simulink model "Quad_Controller"  (R2022b)
settings: Solver=ode4  StartTime=0.0  StopTime=20  FixedStep=0.01  RelTol=1e-3
InitFcn:
  | Initialize
StopFcn:
  | ending
values from neighbouring files (symbols this model uses):
  body =     [Initial_WorkSpace.mat]
  chi0 =     [Initial_WorkSpace.mat]
  g = 9.81    [Initial_WorkSpace.mat]    (also in Initialize.m)
  lambda0 =     [Initial_WorkSpace.mat]
  omega0 =     [Initial_WorkSpace.mat]
  s = tf('s')    [Initialize.m]
  v0 =     [Initial_WorkSpace.mat]
  wh = 250.367142553    [Initial_WorkSpace.mat]    (also in Initialize.m = sqrt(body.m*g/4/body.b))
undefined symbols (not defined in the file or in its folder): X, Y, Z
libraries: nesl_utility x22, sm_lib x17, simulink x5, sharedtransform x4, simulink_extras x3, matrix_library x2, uavutilslib x1
settings Model: Creator=Alire  LastModifiedBy=Alire

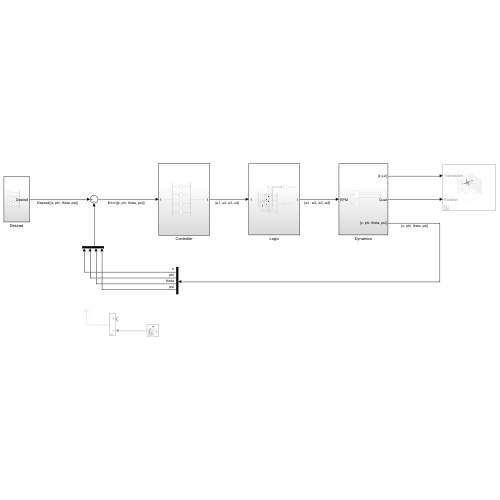
[thumbnail: Simulink's stored preview of the top-level diagram]
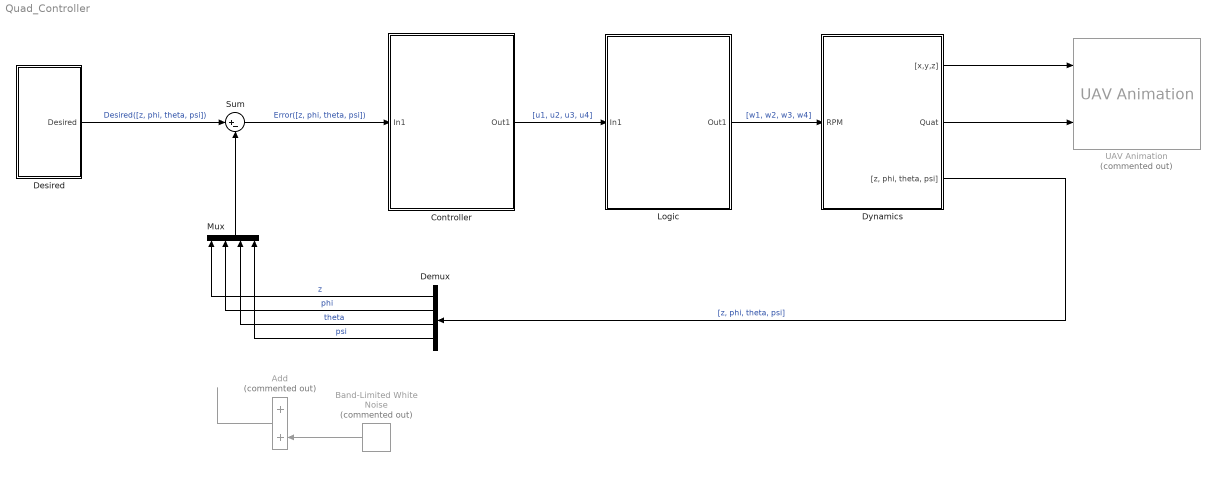
== system Quad_Controller ==
  Add : Sum  Commented=on
  Band-Limited White Noise : simulink/Sources/Band-Limited White Noise  Commented=on  Cov=[0.5*(pi/180)]  Ts=0.1  seed=[23341]
  Controller : Subsystem
  Demux : Demux
  Desired : Subsystem
  Dynamics : Subsystem
  Logic : Subsystem
  Mux : Mux
  Sum : Sum  Inputs=|+-
  UAV Animation : uavutilslib/UAV Animation  Commented=on  UAVType=Multirotor  UAVSize=10  InertialZDirection=Down  SampleTime=-1
  wires:
  Desired/1(Desired) -> Sum/1  "Desired([z, phi, theta, psi])"
  Sum/1 -> Controller/1(In1)  "Error([z, phi, theta, psi])"
  Controller/1(Out1) -> Logic/1(In1)  "[u1, u2, u3, u4]"
  Logic/1(Out1) -> Dynamics/1(RPM)  "[w1, w2, w3, w4]"
  Dynamics/3("[z, phi, theta, psi]") -> Demux/1  "[z, phi, theta, psi]"
  Dynamics/1("[x,y,z]") -> UAV Animation/1
  Dynamics/2(Quat) -> UAV Animation/2
  Mux/1 -> Sum/2
  Demux/1 -> Mux/1  "z"
  Demux/2 -> Mux/2  "phi"
  Demux/3 -> Mux/3  "theta"
  Demux/4 -> Mux/4  "psi"
  Band-Limited White Noise/1 -> Add/2
  Add/1 -> ?

== system Quad_Controller/Controller ==
  In1 : Inport
  Demux : Demux
  Gc_phi : Subsystem
  Gc_psi : Subsystem
  Gc_theta : Subsystem
  Gc_z : Subsystem
  Mux : Mux
  Out1 : Outport
  wires:
  In1/1 -> Demux/1
  Mux/1 -> Out1/1
  Demux/1 -> Gc_z/1(In1)
  Gc_z/1(u1) -> Mux/1
  Demux/2 -> Gc_phi/1(In1)
  Demux/3 -> Gc_theta/1(In1)
  Gc_theta/1(u3) -> Mux/3
  Gc_psi/1(u4) -> Mux/4
  Demux/4 -> Gc_psi/1(In1)
  Gc_phi/1(u2) -> Mux/2

== system Quad_Controller/Desired ==
  Degrees to Radians : simulink_extras/Transformations/Degrees to Radians
  Degrees to Radians1 : simulink_extras/Transformations/Degrees to Radians
  Degrees to Radians2 : simulink_extras/Transformations/Degrees to Radians
  Mux : Mux
  Z_desired : Constant  Value=-1
  phi_desired : Constant  Value=0
  psi_desired : Constant  Value=8
  theta_desired : Constant  Value=0
  Desired : Outport
  wires:
  Z_desired/1 -> Mux/1
  Mux/1 -> Desired/1
  theta_desired/1 -> Degrees to Radians1/1
  phi_desired/1 -> Degrees to Radians/1
  psi_desired/1 -> Degrees to Radians2/1
  Degrees to Radians/1 -> Mux/2
  Degrees to Radians1/1 -> Mux/3
  Degrees to Radians2/1 -> Mux/4

== system Quad_Controller/Dynamics ==
  RPM : Inport
  Phase1_Model : Subsystem
  Phase3_Model : Subsystem  Commented=on
  "[x,y,z]" : Outport
  Quat : Outport  Port=2
  "[z, phi, theta, psi]" : Outport  Port=3
  wires:
  RPM/1 -> Phase3_Model/1(rpm), Phase1_Model/1(RPM)
  Phase1_Model/1(x,y,z) -> "[x,y,z]"/1
  Phase1_Model/2(Quat) -> Quat/1
  Phase1_Model/3("[z, lambda]") -> "[z, phi, theta, psi]"/1

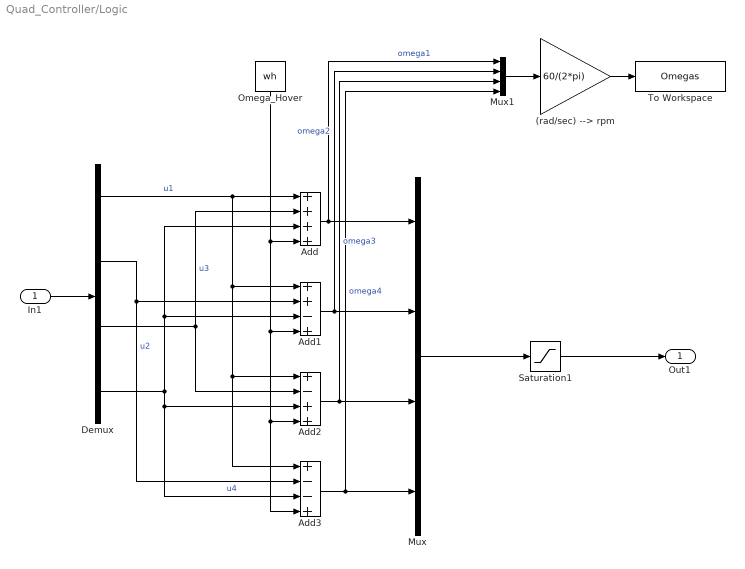
== system Quad_Controller/Logic ==
  In1 : Inport
  (rad/sec) --> rpm : Gain  Gain=60/(2*pi)
  Add : Sum  Inputs=++++
  Add1 : Sum  Inputs=++-+
  Add2 : Sum  Inputs=+-++
  Add3 : Sum  Inputs=+--+
  Demux : Demux
  Mux : Mux
  Mux1 : Mux
  Omega_Hover : Constant  Value=wh
  Saturation1 : Saturate  UpperLimit=350  LowerLimit=-200
  To Workspace : ToWorkspace  VariableName=Omegas  SampleTime=-1
  Out1 : Outport
  wires:
  In1/1 -> Demux/1
  Demux/1 -> Add/1, Add3/1, Add2/1, Add1/1  "u1"
  Demux/2 -> Add3/2, Add1/2  "u2"
  Demux/3 -> Add2/2, Add/2  "u3"
  Demux/4 -> Add2/3, Add3/3, Add1/3, Add/3  "u4"
  Add/1 -> Mux/1, Mux1/1  "omega1"
  Add1/1 -> Mux/2, Mux1/2  "omega2"
  Add2/1 -> Mux/3, Mux1/3  "omega3"
  Add3/1 -> Mux/4, Mux1/4  "omega4"
  Mux/1 -> Saturation1/1
  Omega_Hover/1 -> Add/4, Add3/4, Add2/4, Add1/4
  Mux1/1 -> (rad/sec) --> rpm/1
  (rad/sec) --> rpm/1 -> To Workspace/1
  Saturation1/1 -> Out1/1

== system Quad_Controller/Controller/Gc_phi ==
  In1 : Inport
  Add : Sum
  Derivative : Derivative
  Gain : Gain  Gain=8.7e3
  Gain1 : Gain  Gain=450
  u2 : Outport
  wires:
  Gain1/1 -> Derivative/1
  Gain/1 -> Add/1
  Add/1 -> u2/1  "u2"
  Derivative/1 -> Add/2
  In1/1 -> Gain/1, Gain1/1

== system Quad_Controller/Controller/Gc_psi ==
  In1 : Inport
  Add : Sum
  Derivative : Derivative
  Gain : Gain  Gain=12.5e3
  Gain1 : Gain  Gain=650
  u4 : Outport
  wires:
  Gain1/1 -> Derivative/1
  Gain/1 -> Add/1
  Add/1 -> u4/1  "u4"
  Derivative/1 -> Add/2
  In1/1 -> Gain1/1, Gain/1

== system Quad_Controller/Controller/Gc_theta ==
  In1 : Inport
  Add : Sum
  Derivative : Derivative
  Gain : Gain  Gain=8.6e3
  Gain1 : Gain  Gain=445
  u3 : Outport
  wires:
  In1/1 -> Gain1/1, Gain/1
  Derivative/1 -> Add/2
  Add/1 -> u3/1  "u3"
  Gain/1 -> Add/1
  Gain1/1 -> Derivative/1

== system Quad_Controller/Controller/Gc_z ==
  In1 : Inport
  Add : Sum
  Derivative : Derivative
  Gain : Gain  Gain=-38e3
  Gain1 : Gain  Gain=-20e3
  u1 : Outport
  wires:
  In1/1 -> Gain1/1, Gain/1
  Derivative/1 -> Add/2
  Add/1 -> u1/1  "u1"
  Gain/1 -> Add/1
  Gain1/1 -> Derivative/1

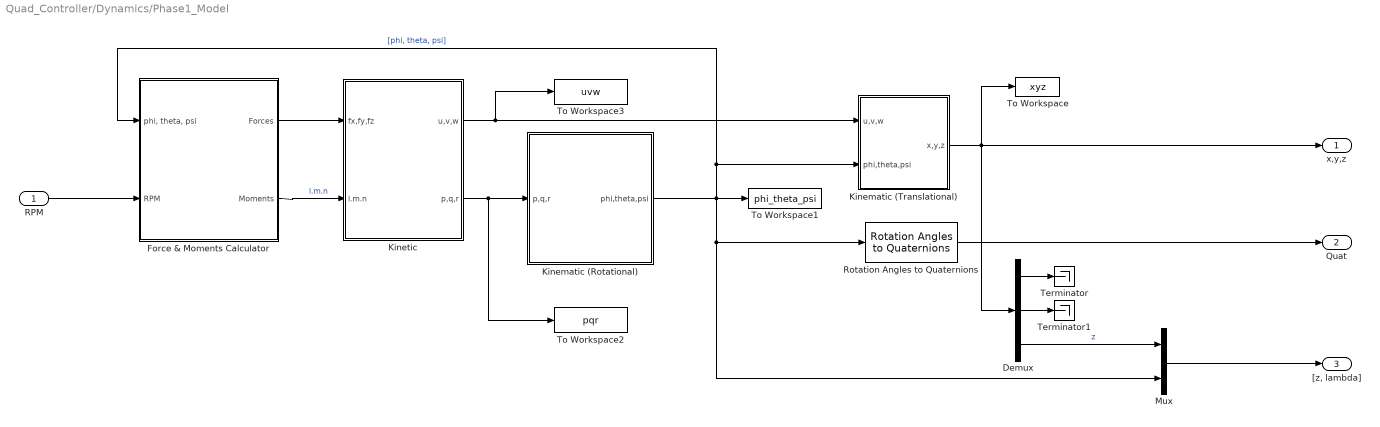
== system Quad_Controller/Dynamics/Phase1_Model ==
  RPM : Inport
  Demux : Demux  Outputs=3
  Force & Moments Calculator : Subsystem
  Kinematic (Rotational) : Subsystem
  Kinematic (Translational) : Subsystem
  Kinetic : Subsystem
  Mux : Mux  Inputs=2
  Rotation Angles to Quaternions : sharedtransform/Rotation Angles to Quaternions  rotationOrder=ZYX  aMode=aMode
  Terminator : Terminator
  Terminator1 : Terminator
  To Workspace : ToWorkspace  VariableName=xyz  SampleTime=-1
  To Workspace1 : ToWorkspace  VariableName=phi_theta_psi  SampleTime=-1
  To Workspace2 : ToWorkspace  VariableName=pqr  SampleTime=-1
  To Workspace3 : ToWorkspace  VariableName=uvw  SampleTime=-1
  x,y,z : Outport
  Quat : Outport  Port=2
  "[z, lambda]" : Outport  Port=3
  wires:
  Kinetic/1(u,v,w) -> Kinematic (Translational)/1(u,v,w), To Workspace3/1
  Kinetic/2(p,q,r) -> To Workspace2/1, Kinematic (Rotational)/1(p,q,r)
  Demux/3 -> Mux/1  "z"
  Force & Moments Calculator/1(Forces) -> Kinetic/1(fx,fy,fz)
  RPM/1 -> Force & Moments Calculator/2(RPM)
  Kinematic (Translational)/1(x,y,z) -> x,y,z/1, Demux/1, To Workspace/1
  Force & Moments Calculator/2(Moments) -> Kinetic/2(l.m.n)  "l.m.n"
  Demux/2 -> Terminator1/1
  Demux/1 -> Terminator/1
  Rotation Angles to Quaternions/1 -> Quat/1
  Kinematic (Rotational)/1(phi,theta,psi) -> Force & Moments Calculator/1("phi, theta, psi"), Kinematic (Translational)/2(phi,theta,psi), Mux/2, Rotation Angles to Quaternions/1, To Workspace1/1  "[phi, theta, psi]"
  Mux/1 -> "[z, lambda]"/1

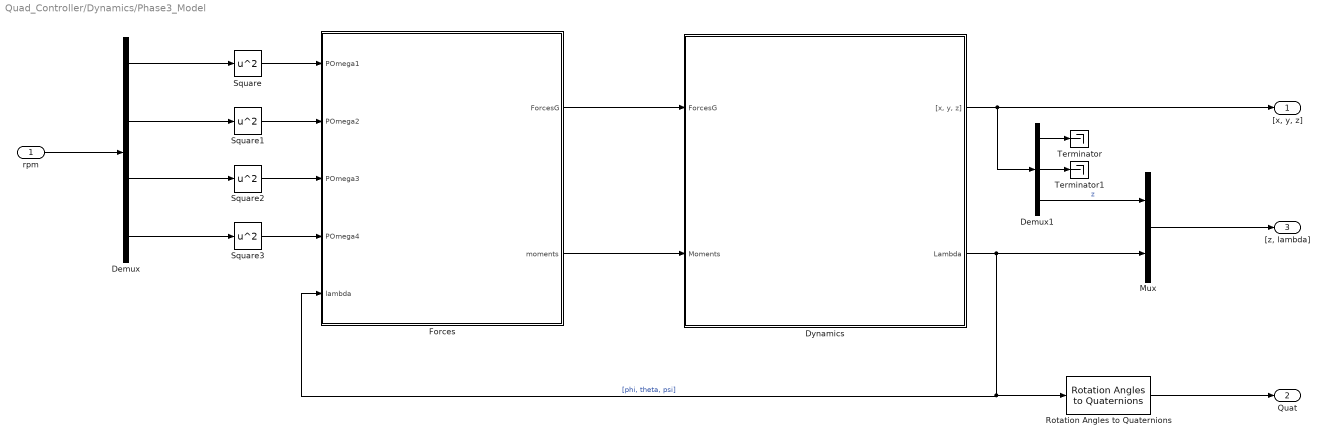
== system Quad_Controller/Dynamics/Phase3_Model ==
  rpm : Inport
  Demux : Demux
  Demux1 : Demux  Outputs=3
  Dynamics : Subsystem
  Forces : Subsystem
  Mux : Mux  Inputs=2
  Rotation Angles to Quaternions : sharedtransform/Rotation Angles to Quaternions  rotationOrder=ZYX  aMode=aMode
  Square{,1..3} (4 alike) : Math  Operator=square
  Terminator : Terminator
  Terminator1 : Terminator
  "[x, y, z]" : Outport
  Quat : Outport  Port=2
  "[z, lambda]" : Outport  Port=3
  wires:
  Demux/1 -> Square/1
  Dynamics/2(Lambda) -> Forces/5(lambda), Rotation Angles to Quaternions/1, Mux/2  "[phi, theta, psi]"
  Square2/1 -> Forces/3(POmega3)
  Square/1 -> Forces/1(POmega1)
  Demux/3 -> Square2/1
  Square1/1 -> Forces/2(POmega2)
  Square3/1 -> Forces/4(POmega4)
  Demux/4 -> Square3/1
  Demux/2 -> Square1/1
  Forces/1(ForcesG) -> Dynamics/1(ForcesG)
  Forces/2(moments) -> Dynamics/2(Moments)
  rpm/1 -> Demux/1
  Mux/1 -> "[z, lambda]"/1
  Demux1/2 -> Terminator1/1
  Demux1/3 -> Mux/1  "z"
  Demux1/1 -> Terminator/1
  Dynamics/1("[x, y, z]") -> "[x, y, z]"/1, Demux1/1
  Rotation Angles to Quaternions/1 -> Quat/1

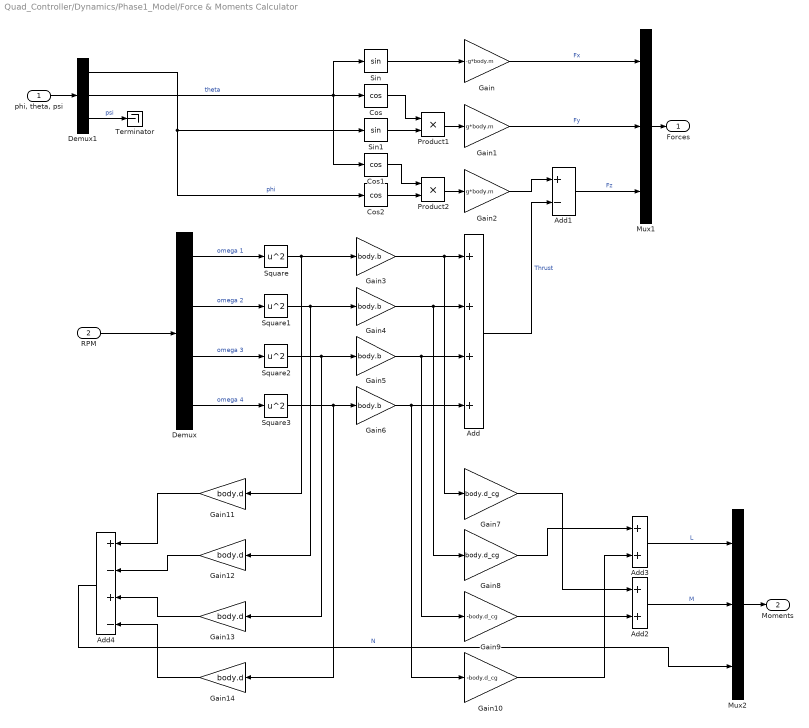
== system Quad_Controller/Dynamics/Phase1_Model/Force & Moments Calculator ==
  "phi, theta, psi" : Inport
  RPM : Inport  Port=2
  Add : Sum  Inputs=++++
  Add1 : Sum  Inputs=+-
  Add2 : Sum
  Add3 : Sum
  Add4 : Sum  Inputs=+-+-
  Cos : Trigonometry  Operator=cos
  Cos1 : Trigonometry  Operator=cos
  Cos2 : Trigonometry  Operator=cos
  Demux : Demux
  Demux1 : Demux  Outputs=3
  Gain : Gain  Gain=-g*body.m
  Gain1 : Gain  Gain=g*body.m
  Gain10 : Gain  Gain=-body.d_cg
  Gain{11..14} (4 alike) : Gain  Gain=body.d
  Gain2 : Gain  Gain=g*body.m
  Gain{3..6} (4 alike) : Gain  Gain=body.b
  Gain7 : Gain  Gain=body.d_cg
  Gain8 : Gain  Gain=body.d_cg
  Gain9 : Gain  Gain=-body.d_cg
  Mux1 : Mux  Inputs=3
  Mux2 : Mux  Inputs=3
  Product1 : Product
  Product2 : Product
  Sin : Trigonometry
  Sin1 : Trigonometry
  Square{,1..3} (4 alike) : Math  Operator=square
  Terminator : Terminator
  Forces : Outport
  Moments : Outport  Port=2
  wires:
  Cos2/1 -> Product2/2
  Cos1/1 -> Product2/1
  Gain1/1 -> Mux1/2  "Fy"
  Demux/3 -> Square2/1  "omega 3"
  Gain5/1 -> Gain9/1, Add/3
  Gain2/1 -> Add1/1
  Demux1/1 -> Sin1/1, Cos2/1  "phi"
  Add3/1 -> Mux2/1  "L"
  Gain4/1 -> Gain8/1, Add/2
  Gain6/1 -> Gain10/1, Add/4
  Gain3/1 -> Gain7/1, Add/1
  Demux/2 -> Square1/1  "omega 2"
  Gain9/1 -> Add2/2
  Sin1/1 -> Product1/2
  Gain/1 -> Mux1/1  "Fx"
  Add2/1 -> Mux2/2  "M"
  Gain13/1 -> Add4/3
  Demux/1 -> Square/1  "omega 1"
  Square2/1 -> Gain13/1, Gain5/1
  Demux1/2 -> Sin/1, Cos1/1, Cos/1  "theta"
  Gain7/1 -> Add2/1
  Gain14/1 -> Add4/4
  Demux/4 -> Square3/1  "omega 4"
  Cos/1 -> Product1/1
  Gain12/1 -> Add4/2
  Square3/1 -> Gain14/1, Gain6/1
  Add/1 -> Add1/2  "Thrust"
  Add4/1 -> Mux2/3  "N"
  Mux2/1 -> Moments/1
  Gain11/1 -> Add4/1
  Sin/1 -> Gain/1
  Product1/1 -> Gain1/1
  Add1/1 -> Mux1/3  "Fz"
  Gain8/1 -> Add3/1
  RPM/1 -> Demux/1
  Square1/1 -> Gain12/1, Gain4/1
  Square/1 -> Gain11/1, Gain3/1
  Gain10/1 -> Add3/2
  Product2/1 -> Gain2/1
  Mux1/1 -> Forces/1
  "phi, theta, psi"/1 -> Demux1/1
  Demux1/3 -> Terminator/1  "psi"

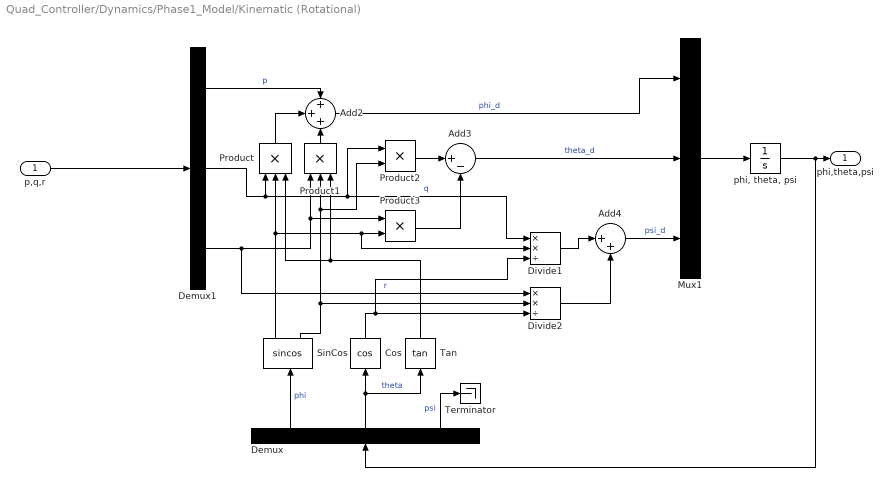
== system Quad_Controller/Dynamics/Phase1_Model/Kinematic (Rotational) ==
  p,q,r : Inport
  Add2 : Sum  Inputs=+++
  Add3 : Sum  Inputs=|+-
  Add4 : Sum  Inputs=|++
  Cos : Trigonometry  Operator=cos
  Demux : Demux  Outputs=3
  Demux1 : Demux  Outputs=3
  Divide1 : Product  Inputs=**/
  Divide2 : Product  Inputs=**/
  Mux1 : Mux  Inputs=3
  Product : Product  Inputs=3
  Product1 : Product  Inputs=3
  Product2 : Product
  Product3 : Product
  SinCos : Trigonometry  Operator=sincos
  Tan : Trigonometry  Operator=tan
  Terminator : Terminator
  "phi, theta, psi" : Integrator  InitialCondition=[lambda0.phi, lambda0.theta, lambda0.psi]
  phi,theta,psi : Outport
  wires:
  SinCos/2 -> Divide2/2, Product2/2, Product1/2
  Divide1/1 -> Add4/1
  Product1/1 -> Add2/3
  Demux1/2 -> Product/1, Divide1/1, Product2/1  "q"
  Demux1/3 -> Divide2/1, Product3/1, Product1/1  "r"
  Product2/1 -> Add3/1
  Tan/1 -> Product1/3, Product/3
  Demux/3 -> Terminator/1  "psi"
  Mux1/1 -> "phi, theta, psi"/1
  Cos/1 -> Divide2/3, Divide1/3
  Demux/1 -> SinCos/1  "phi"
  SinCos/1 -> Divide1/2, Product3/2, Product/2
  Add2/1 -> Mux1/1  "phi_d"
  Demux1/1 -> Add2/1  "p"
  Product/1 -> Add2/2
  Demux/2 -> Cos/1, Tan/1  "theta"
  Product3/1 -> Add3/2
  Add3/1 -> Mux1/2  "theta_d"
  Add4/1 -> Mux1/3  "psi_d"
  Divide2/1 -> Add4/2
  "phi, theta, psi"/1 -> Demux/1, phi,theta,psi/1
  p,q,r/1 -> Demux1/1

== system Quad_Controller/Dynamics/Phase1_Model/Kinematic (Translational) ==
  u,v,w : Inport
  phi,theta,psi : Inport  Port=2
  MatrixMultiply2 : Product  Multiplication=Matrix(*)
  Rotation Angles to Direction Cosine Matrix : sharedtransform/Rotation Angles to Direction Cosine Matrix  rotationOrder=ZYX  aMode=aMode
  Selector9 : Selector  InputPortWidth=3  IndexOptions=Index vector (dialog)  Indices=[3 2 1]  OutputSizes=1
  Transpose : Math  Operator=transpose
  "x, y, z" : Integrator  InitialCondition=[chi0.x, chi0.y, chi0.z]
  x,y,z : Outport
  wires:
  Transpose/1 -> MatrixMultiply2/1
  Selector9/1 -> Rotation Angles to Direction Cosine Matrix/1
  MatrixMultiply2/1 -> "x, y, z"/1
  u,v,w/1 -> MatrixMultiply2/2
  Rotation Angles to Direction Cosine Matrix/1 -> Transpose/1
  "x, y, z"/1 -> x,y,z/1
  phi,theta,psi/1 -> Selector9/1

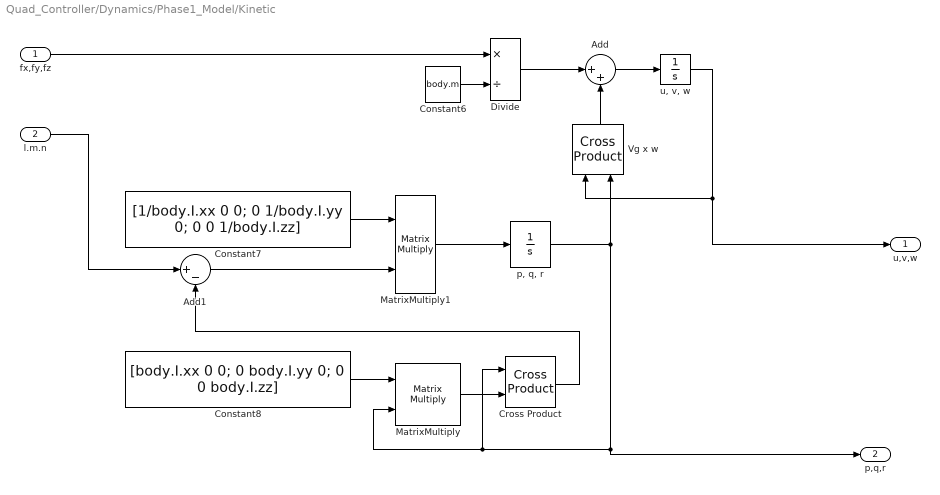
== system Quad_Controller/Dynamics/Phase1_Model/Kinetic ==
  fx,fy,fz : Inport
  l.m.n : Inport  Port=2
  Add : Sum  Inputs=|++
  Add1 : Sum  Inputs=|+-
  Constant6 : Constant  Value=body.m
  Constant7 : Constant  Value="[1/body.I.xx 0 0; 0 1/body.I.yy 0; 0 0  1/body.I.zz]"
  Constant8 : Constant  Value="[body.I.xx 0 0; 0 body.I.yy 0; 0 0  body.I.zz]"
  Cross Product : matrix_library/Cross Product
  Divide : Product  Inputs=*/
  MatrixMultiply : Product  Multiplication=Matrix(*)
  MatrixMultiply1 : Product  Multiplication=Matrix(*)
  Vg x w : matrix_library/Cross Product
  "p, q, r" : Integrator  InitialCondition=[omega0.p, omega0.q, omega0.r]
  "u, v, w" : Integrator  InitialCondition=[v0.x, v0.y, v0.z]
  u,v,w : Outport
  p,q,r : Outport  Port=2
  wires:
  "u, v, w"/1 -> u,v,w/1, Vg x w/1
  Vg x w/1 -> Add/2
  Constant6/1 -> Divide/2
  Add1/1 -> MatrixMultiply1/2
  "p, q, r"/1 -> p,q,r/1, Cross Product/1, MatrixMultiply/2, Vg x w/2
  Divide/1 -> Add/1
  Constant8/1 -> MatrixMultiply/1
  Add/1 -> "u, v, w"/1
  Cross Product/1 -> Add1/2
  MatrixMultiply/1 -> Cross Product/2
  Constant7/1 -> MatrixMultiply1/1
  fx,fy,fz/1 -> Divide/1
  MatrixMultiply1/1 -> "p, q, r"/1
  l.m.n/1 -> Add1/1

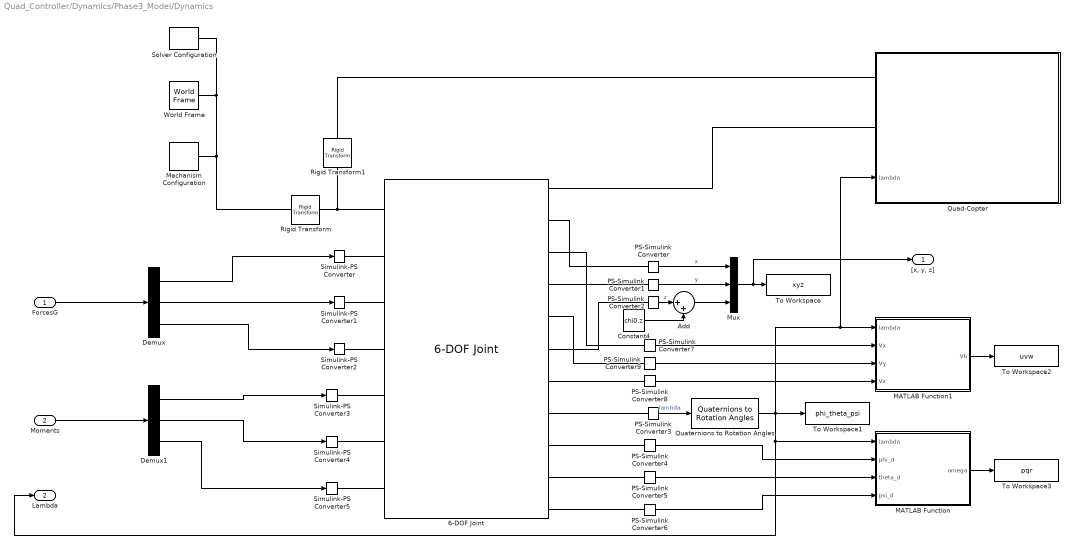
== system Quad_Controller/Dynamics/Phase3_Model/Dynamics ==
  ForcesG : Inport
  Moments : Inport  Port=2
  6-DOF Joint : sm_lib/Joints/6-DOF Joint  JointMode=Normal  SenseConstraintForce=off  SenseConstraintForceX=off  SenseConstraintForceY=off  SenseConstraintForceZ=off  SenseConstraintTorque=off  SenseConstraintTorqueX=off  SenseConstraintTorqueY=off  SenseConstraintTorqueZ=off  SenseTotalForce=off  SenseTotalForceX=off  SenseTotalForceY=off  SenseTotalForceZ=off  SenseTotalTorque=off  SenseTotalTorqueX=off  SenseTotalTorqueY=off  SenseTotalTorqueZ=off  CompositeWrenchDir=FollowerOnBase  CompositeWrenchFrame=BaseFrame  PxEquilibriumPosition=0  PxEquilibriumPositionUnits=m  PxSpringStiffness=0  PxSpringStiffnessUnits=N/m  PxDampingCoefficient=0  PxDampingCoefficientUnits=N/(m/s)  PxTorqueActuationMode=InputTorque  PxMotionActuationMode=ComputedMotion  PxSensePosition=on  PxSenseVelocity=on  PxSenseAcceleration=off  PxSenseTorqueForce=off  PxSenseLowerLimitTorqueForce=off  PxSenseUpperLimitTorqueForce=off  PxLowerLimitSpecify=off  PxLowerLimitBound=-1  PxLowerLimitBoundUnits=m  PxLowerLimitStiffness=1e6  PxLowerLimitStiffnessUnits=N/m  PxLowerLimitDamping=1e3  PxLowerLimitDampingUnits=N/(m/s)  PxLowerLimitTransitionRegionWidth=1e-4  PxLowerLimitTransitionRegionWidthUnits=m  PxUpperLimitSpecify=off  PxUpperLimitBound=1  PxUpperLimitBoundUnits=m  PxUpperLimitStiffness=1e6  PxUpperLimitStiffnessUnits=N/m  PxUpperLimitDamping=1e3  PxUpperLimitDampingUnits=N/(m/s)  PxUpperLimitTransitionRegionWidth=1e-4  PxUpperLimitTransitionRegionWidthUnits=m  PxPositionTargetSpecify=off  PxPositionTargetPriority=High  PxPositionTargetValue=0  PxPositionTargetValueUnits=m  PxVelocityTargetSpecify=off  PxVelocityTargetPriority=High  PxVelocityTargetValue=0  PxVelocityTargetValueUnits=m/s  PyEquilibriumPosition=0  PyEquilibriumPositionUnits=m  PySpringStiffness=0  PySpringStiffnessUnits=N/m  PyDampingCoefficient=0  PyDampingCoefficientUnits=N/(m/s)  PyTorqueActuationMode=InputTorque  PyMotionActuationMode=ComputedMotion  PySensePosition=on  PySenseVelocity=on  PySenseAcceleration=off  PySenseTorqueForce=off  PySenseLowerLimitTorqueForce=off  PySenseUpperLimitTorqueForce=off  PyLowerLimitSpecify=off  PyLowerLimitBound=-1  PyLowerLimitBoundUnits=m  PyLowerLimitStiffness=1e6  PyLowerLimitStiffnessUnits=N/m  PyLowerLimitDamping=1e3  PyLowerLimitDampingUnits=N/(m/s)  PyLowerLimitTransitionRegionWidth=1e-4  PyLowerLimitTransitionRegionWidthUnits=m  PyUpperLimitSpecify=off  PyUpperLimitBound=1  PyUpperLimitBoundUnits=m  PyUpperLimitStiffness=1e6  PyUpperLimitStiffnessUnits=N/m  PyUpperLimitDamping=1e3  PyUpperLimitDampingUnits=N/(m/s)  PyUpperLimitTransitionRegionWidth=1e-4  PyUpperLimitTransitionRegionWidthUnits=m  PyPositionTargetSpecify=off  PyPositionTargetPriority=High  PyPositionTargetValue=0  PyPositionTargetValueUnits=m  PyVelocityTargetSpecify=off  PyVelocityTargetPriority=High  PyVelocityTargetValue=0  PyVelocityTargetValueUnits=m/s  PzEquilibriumPosition=0  PzEquilibriumPositionUnits=m  PzSpringStiffness=0  PzSpringStiffnessUnits=N/m  PzDampingCoefficient=0  PzDampingCoefficientUnits=N/(m/s)  PzTorqueActuationMode=InputTorque  PzMotionActuationMode=ComputedMotion  PzSensePosition=on  PzSenseVelocity=on  PzSenseAcceleration=off  PzSenseTorqueForce=off  PzSenseLowerLimitTorqueForce=off  PzSenseUpperLimitTorqueForce=off  PzLowerLimitSpecify=off  PzLowerLimitBound=-1  PzLowerLimitBoundUnits=m  PzLowerLimitStiffness=1e6  PzLowerLimitStiffnessUnits=N/m  PzLowerLimitDamping=1e3  PzLowerLimitDampingUnits=N/(m/s)  PzLowerLimitTransitionRegionWidth=1e-4  PzLowerLimitTransitionRegionWidthUnits=m  PzUpperLimitSpecify=off  PzUpperLimitBound=1  PzUpperLimitBoundUnits=m  PzUpperLimitStiffness=1e6  PzUpperLimitStiffnessUnits=N/m  PzUpperLimitDamping=1e3  PzUpperLimitDampingUnits=N/(m/s)  PzUpperLimitTransitionRegionWidth=1e-4  PzUpperLimitTransitionRegionWidthUnits=m  PzPositionTargetSpecify=off  PzPositionTargetPriority=High  PzPositionTargetValue=0  PzPositionTargetValueUnits=m  PzVelocityTargetSpecify=off  PzVelocityTargetPriority=High  PzVelocityTargetValue=0  PzVelocityTargetValueUnits=m/s  SphEqPosRotationMethod=None  SphEqPosRotationAngleUnits=deg  SphEqPosRotationStandardAxis=+Z  SphEqPosRotationAngle=0.0  SphEqPosRotationArbitraryAxis=[0 0 1]  SphEqPosFollAlignAxisA=+X  SphEqPosBaseAlignAxisA=+Y  SphEqPosFollAlignAxisB=+Y  SphEqPosBaseAlignAxisB=+Z  SphEqPosRotationSequenceAxes=FollowerAxes  SphEqPosRotationSequence=XYX  SphEqPosRotationSequenceAngles=[0 0 0]  SphEqPosRotationSequenceAnglesUnits=deg  SphEqPosRotationMatrix=[1 0 0; 0 1 0; 0 0 1]  SphEqPosQuaternion=[1 0 0 0]  SphSpringStiffness=0  SphSpringStiffnessUnits=N*m/deg  SphDampingCoefficient=0  SphDampingCoefficientUnits=N*m/(deg/s)  SphActuateTorqueX=on  SphActuateTorqueY=on  SphActuateTorqueZ=on  SphActuateTorque=off  SphTorqueActuationMode=InputTorque  SphMotionActuationMode=ComputedMotion  SphActuationFrame=BaseFrame  SphSensePosition=on  SphSenseVelocityX=on  SphSenseVelocityY=on  SphSenseVelocityZ=on  SphSenseVelocity=off  SphSenseAccelerationX=off  SphSenseAccelerationY=off  SphSenseAccelerationZ=off  SphSenseAcceleration=off  SphSenseTorqueX=off  SphSenseTorqueY=off  SphSenseTorqueZ=off  SphSenseTorqueForce=off  SphSenseLowerLimitTorqueMag=off  SphSenseUpperLimitTorqueMag=off  SphSensingFrame=BaseFrame  SphLowerLimitSpecify=off  SphLowerLimitBound=15  SphLowerLimitBoundUnits=deg  SphLowerLimitStiffness=1e4  SphLowerLimitStiffnessUnits=N*m/deg  SphLowerLimitDamping=10  SphLowerLimitDampingUnits=N*m/(deg/s)  SphLowerLimitTransitionRegionWidth=0.1  SphLowerLimitTransitionRegionWidthUnits=deg  SphUpperLimitSpecify=off  SphUpperLimitBound=45  SphUpperLimitBoundUnits=deg  SphUpperLimitStiffness=1e4  SphUpperLimitStiffnessUnits=N*m/deg  SphUpperLimitDamping=10  SphUpperLimitDampingUnits=N*m/(deg/s)  SphUpperLimitTransitionRegionWidth=0.1  SphUpperLimitTransitionRegionWidthUnits=deg  SphPositionTargetRotationMethod=None  SphPositionTargetRotationAngleUnits=deg  SphPositionTargetRotationStandardAxis=+Z  SphPositionTargetRotationAngle=0.0  SphPositionTargetRotationArbitraryAxis=[0 0 1]  SphPositionTargetFollAlignAxisA=+X  SphPositionTargetBaseAlignAxisA=+Y  SphPositionTargetFollAlignAxisB=+Y  SphPositionTargetBaseAlignAxisB=+Z  SphPositionTargetRotationSequenceAxes=FollowerAxes  SphPositionTargetRotationSequence=XYX  SphPositionTargetRotationSequenceAngles=[0 0 0]  SphPositionTargetRotationSequenceAnglesUnits=deg  SphPositionTargetRotationMatrix=[1 0 0; 0 1 0; 0 0 1]  SphPositionTargetQuaternion=[1 0 0 0]  SphPositionTargetSpecify=off  SphPositionTargetPriority=High  SphVelocityTargetValue=[0 0 0]  SphVelocityTargetValueUnits=deg/s  SphVelocityTargetSpecify=off  SphVelocityTargetPriority=High  SphVelocityTargetInFollowerFrame=on
  Add : Sum  Inputs=|++
  Constant4 : Constant  Value=chi0.z
  Demux : Demux  Outputs=3
  Demux1 : Demux  Outputs=3
  MATLAB Function : MATLAB Function  TreatAsAtomicUnit=on
  MATLAB Function1 : MATLAB Function  TreatAsAtomicUnit=on
  Mechanism Configuration : sm_lib/Utilities/Mechanism Configuration  UniformGravity=Constant  GravityVector=[0 0 -9.81]  GravityUnits=m/s^2  LinearizationDelta=0.001  JointModeTransitionNonlinearIterations=2
  Mux : Mux  Inputs=3
  PS-Simulink Converter{,1..9} (10 alike) : nesl_utility/PS-Simulink Converter  PhysicalDomain=network_engine_domain  SubClassName=ps_output  LeftPortType=input  RightPortType=output  PseudoPeriodic=off  Frequencies=[]  VectorFormat=inherit  Unit=inherit  AffineConversion=off
  Quad-Copter : Subsystem
      settings: PortSchema="{\"entries\":[{\"content\":{\"sides\":[{\"content\":{\"connectorIds\":[\"LConn1\",\"LConn2\",\"In1\"]},\"type\":\"ConnectorPlacement.EquallySpacedRectSide\",\"uuid\":\"04743956-a569-41a7-b22c-bd483dcea0b7\"},{\"content\":{\"connectorIds\":[],\"side\":\"RIGHT\"},\"type\":\"ConnectorPlacement.EquallySpacedRectSide\",\"uuid\":\"9bc8017a-87dc-4fac-922f-a31a079728db\"},{\"content\":{\"connectorIds\":[],\"side\":\"TOP\"},\"type\":\"ConnectorPlacement.EquallySpacedRectSide\",\"uuid\":\"e9bdb144-97c5-4666-a0dc-c713dd3d3caa\"}]},\"type\":\"ConnectorPlacement.EquallySpacedConnector\",\"uuid\":\"315c4317-d40d-4cb5-b79a-0df11d629229\"}],\"packageUris\":[\"http://schema.mathworks.com/mf0/Connector/R2020b\"],\"version\":\"1.0\"}"
  Quaternions to Rotation Angles : sharedtransform/Quaternions to Rotation Angles  rotationOrder=XYZ  aMode=aMode
  Rigid Transform : sm_lib/Frames and Transforms/Rigid Transform  TranslationMethod=None  TranslationStandardOffset=0  TranslationLengthUnit=m  TranslationStandardAxis=+Z  TranslationCartesianOffset=[0 0 0]  TranslationROffset=0  TranslationROffsetUnits=m  TranslationZOffset=0  TranslationZOffsetUnits=m  TranslationThetaOffset=0  TranslationThetaOffsetUnits=deg  RotationMethod=StandardAxis  RotationAngleUnits=deg  RotationStandardAxis=+X  RotationAngle=180  RotationArbitraryAxis=[0 0 1]  FollAlignAxisA=+X  BaseAlignAxisA=+Y  FollAlignAxisB=+Y  BaseAlignAxisB=+Z  RotationSequenceAxes=FollowerAxes  RotationSequence=XYX  RotationSequenceAngles=[0 0 0]  RotationSequenceAnglesUnits=deg  RotationMatrix=[1 0 0; 0 1 0; 0 0 1]  Quaternion=[1 0 0 0]
  Rigid Transform1 : sm_lib/Frames and Transforms/Rigid Transform  TranslationMethod=StandardAxis  TranslationStandardOffset=1  TranslationLengthUnit=m  TranslationStandardAxis=+Z  TranslationCartesianOffset=[0 0 0]  TranslationROffset=0  TranslationROffsetUnits=m  TranslationZOffset=0  TranslationZOffsetUnits=m  TranslationThetaOffset=0  TranslationThetaOffsetUnits=deg  RotationMethod=None  RotationAngleUnits=deg  RotationStandardAxis=+X  RotationAngle=180  RotationArbitraryAxis=[0 0 1]  FollAlignAxisA=+X  BaseAlignAxisA=+Y  FollAlignAxisB=+Y  BaseAlignAxisB=+Z  RotationSequenceAxes=FollowerAxes  RotationSequence=XYX  RotationSequenceAngles=[0 0 0]  RotationSequenceAnglesUnits=deg  RotationMatrix=[1 0 0; 0 1 0; 0 0 1]  Quaternion=[1 0 0 0]
  Simulink-PS Converter{,1..5} (6 alike) : nesl_utility/Simulink-PS Converter  PhysicalDomain=network_engine_domain  SubClassName=ps_input  LeftPortType=input  RightPortType=output  PseudoPeriodic=off  Frequencies=[]  NoiseDistribution=none  NoiseParameters=[]  Unit=1  AffineConversion=off  FilteringAndDerivatives=provide  SimscapeFilterOrder=1  InputFilterTimeConstant=0.001  UdotUserProvided=0
  Solver Configuration : nesl_utility/Solver Configuration  PhysicalDomain=network_engine_domain  SubClassName=solver  LeftPortType=input  RightPortType=generic  Tones=[]  Harmonics=[]  SimulateNoise=off  Profile=off  UseLocalSampling=off  EnableSwitchedLinearOptims=on  FrequencyDomain=off  UseCCode=off  RelTol=0.001  AbsTol=1e-06  MinStep=1e-09  ToWorkspace=off  RevertToSquareIcSolve=off  NumHomotopyIterations=100  PhasorMode=off  PhasorModeNumHarmonics=1  ConsistencySolver=NEWTON_XTOL_AFTER_FTOL  IndexReductionMethod=DerivativeReplacement  DoDC=off  ResidualTolerance=1e-09  ConsistencyTolSource=GLOBAL  ConsistencyAbsTol=0.001  ConsistencyRelTol=0.001  ConsistencyTolFactor=0.001  UseLocalSolver=off  LocalSolverChoice=NE_BACKWARD_EULER_ADVANCER  ResolveIndetEquations=on  FunctionEvalNumThread=1  LocalSolverSampleTime=0.001  DoFixedCost=off  MaxNonlinIter=3  MaxModeIter=2  ComputeImpulses=off  ImpulseIterations=2  LinearAlgebra=Sparse  LinearAlgebraNumThread=0  EquationFormulation=NE_TIME_EF  DelaysMemoryBudget=1024  AutomaticFiltering=on  FilteringTimeConstant=0.001  PartitionStorageMethod=AS_NEEDED  PartitionMemoryBudget=1024  PartitionMethod=FAST
  To Workspace : ToWorkspace  VariableName=xyz  SampleTime=-1
      settings: Save2DSignal=2-D array (concatenate along first dimension)
  To Workspace1 : ToWorkspace  VariableName=phi_theta_psi  SampleTime=-1
      settings: Save2DSignal=2-D array (concatenate along first dimension)
  To Workspace2 : ToWorkspace  VariableName=uvw  SampleTime=-1
      settings: Save2DSignal=2-D array (concatenate along first dimension)
  To Workspace3 : ToWorkspace  VariableName=pqr  SampleTime=-1
      settings: Save2DSignal=2-D array (concatenate along first dimension)
  World Frame : sm_lib/Frames and Transforms/World Frame
  "[x, y, z]" : Outport
  Lambda : Outport  Port=2
  wires:
  PS-Simulink Converter/1 -> Mux/1  "x"
  PS-Simulink Converter9/1 -> MATLAB Function1/3(Vy)
  Add/1 -> Mux/3
  Demux/2 -> Simulink-PS Converter1/1
  PS-Simulink Converter2/1 -> Add/1  "z"
  Quaternions to Rotation Angles/1 -> Quad-Copter/1(lambda), MATLAB Function1/1(lambda), Lambda/1, MATLAB Function/1(lambda), To Workspace1/1
  Demux1/1 -> Simulink-PS Converter3/1
  Demux/3 -> Simulink-PS Converter2/1
  ForcesG/1 -> Demux/1
  PS-Simulink Converter1/1 -> Mux/2  "y"
  PS-Simulink Converter8/1 -> MATLAB Function1/4(Vz)
  Demux1/3 -> Simulink-PS Converter5/1
  PS-Simulink Converter5/1 -> MATLAB Function/3(theta_d)
  Demux1/2 -> Simulink-PS Converter4/1
  Constant4/1 -> Add/2
  Demux/1 -> Simulink-PS Converter/1
  Mux/1 -> "[x, y, z]"/1, To Workspace/1
  MATLAB Function/1(omega) -> To Workspace3/1
  PS-Simulink Converter4/1 -> MATLAB Function/2(phi_d)
  PS-Simulink Converter3/1 -> Quaternions to Rotation Angles/1  "lambda"
  MATLAB Function1/1(Vb) -> To Workspace2/1
  PS-Simulink Converter7/1 -> MATLAB Function1/2(Vx)
  PS-Simulink Converter6/1 -> MATLAB Function/4(psi_d)
  Moments/1 -> Demux1/1
  connections:
  Rigid Transform/RConn1 -- 6-DOF Joint/LConn1 -- Rigid Transform1/LConn1
  Simulink-PS Converter1/RConn1 -- 6-DOF Joint/LConn3
  6-DOF Joint/RConn2 -- PS-Simulink Converter/LConn1
  Simulink-PS Converter2/RConn1 -- 6-DOF Joint/LConn4
  PS-Simulink Converter1/LConn1 -- 6-DOF Joint/RConn4
  6-DOF Joint/RConn11 -- PS-Simulink Converter6/LConn1
  6-DOF Joint/RConn8 -- PS-Simulink Converter3/LConn1
  6-DOF Joint/RConn6 -- PS-Simulink Converter2/LConn1
  6-DOF Joint/RConn10 -- PS-Simulink Converter5/LConn1
  6-DOF Joint/RConn5 -- PS-Simulink Converter9/LConn1
  Mechanism Configuration/RConn1 -- Rigid Transform/LConn1 -- World Frame/RConn1 -- Solver Configuration/RConn1
  Simulink-PS Converter5/RConn1 -- 6-DOF Joint/LConn7
  Simulink-PS Converter/RConn1 -- 6-DOF Joint/LConn2
  Simulink-PS Converter4/RConn1 -- 6-DOF Joint/LConn6
  6-DOF Joint/RConn7 -- PS-Simulink Converter8/LConn1
  Simulink-PS Converter3/RConn1 -- 6-DOF Joint/LConn5
  6-DOF Joint/RConn9 -- PS-Simulink Converter4/LConn1
  6-DOF Joint/RConn3 -- PS-Simulink Converter7/LConn1
  Quad-Copter/LConn2 -- 6-DOF Joint/RConn1
  Rigid Transform1/RConn1 -- Quad-Copter/LConn1

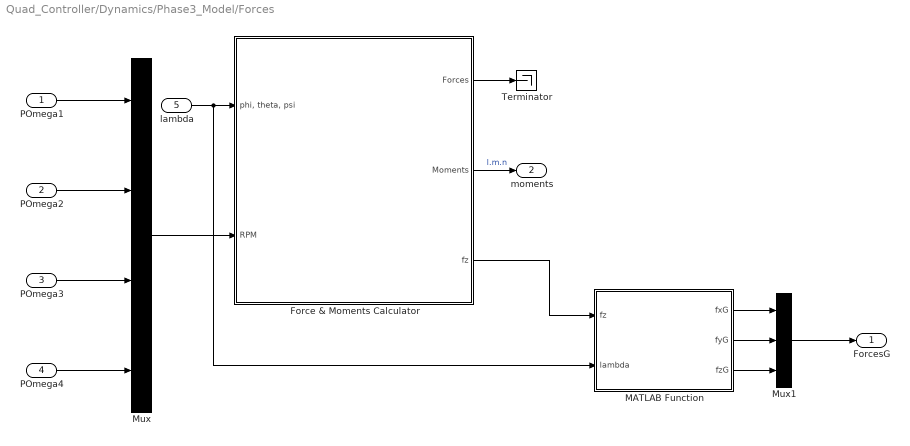
== system Quad_Controller/Dynamics/Phase3_Model/Forces ==
  POmega1 : Inport
  POmega2 : Inport  Port=2
  POmega3 : Inport  Port=3
  POmega4 : Inport  Port=4
  lambda : Inport  Port=5
  Force & Moments Calculator : Subsystem
  MATLAB Function : MATLAB Function  TreatAsAtomicUnit=on
  Mux : Mux
  Mux1 : Mux  Inputs=3
  Terminator : Terminator
  ForcesG : Outport
  moments : Outport  Port=2
  wires:
  Force & Moments Calculator/2(Moments) -> moments/1  "l.m.n"
  POmega3/1 -> Mux/3
  POmega1/1 -> Mux/1
  Mux/1 -> Force & Moments Calculator/2(RPM)
  POmega4/1 -> Mux/4
  POmega2/1 -> Mux/2
  lambda/1 -> MATLAB Function/2(lambda), Force & Moments Calculator/1("phi, theta, psi")
  Force & Moments Calculator/3(fz) -> MATLAB Function/1(fz)
  MATLAB Function/1(fxG) -> Mux1/1
  MATLAB Function/2(fyG) -> Mux1/2
  MATLAB Function/3(fzG) -> Mux1/3
  Mux1/1 -> ForcesG/1
  Force & Moments Calculator/1(Forces) -> Terminator/1

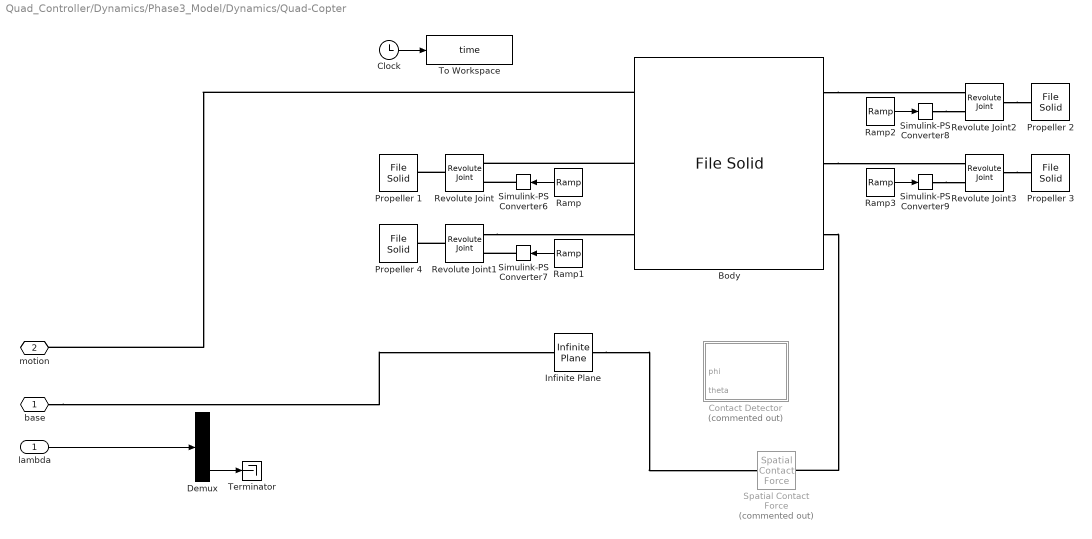
== system Quad_Controller/Dynamics/Phase3_Model/Dynamics/Quad-Copter ==
  lambda : Inport
  Body : sm_lib/Body Elements/File Solid  ExtGeomFileName=SolidFiles\body.STEP  UnitType=FromFile  ExtGeomFileUnits=m  StepReaderType=HEX  ExportConvexHullGeometry=on  InertiaType=Custom  Mass=0.8  MassUnits=kg  CenterOfMass=[-333.85 324.3 -438.13]  CenterOfMassUnits=mm  MomentsOfInertia=[0.02839 0.03066 0.04390]  MomentsOfInertiaUnits=kg*m^2  ProductsOfInertia=[0 0 0]  ProductsOfInertiaUnits=kg*m^2  BasedOnType=DensityFromFile  Density=1000  DensityUnits=kg/m^3  DoExposeReferenceFrame=off  SerializedFrames=<Frames><Frame><Id>Frame1</Id><Value><Name>CG</Name><Origin><Source>CenterOfMassFrame</Source><FeatureName></FeatureName></Origin><PrimaryAxis><DefinedDirection>+Z</DefinedDirection><Source>ReferenceFrame</Source><SourceDirection>+Z</SourceDirection><FeatureName></FeatureName></PrimaryAxis><SecondaryAxis><DefinedDirection>+X</DefinedDirection><Source>ReferenceFrame</Source><SourceDirection>+X</SourceDirection><FeatureName></FeatureName></SecondaryAxis></Value></Frame><Frame><Id>Frame2</Id><Value><Name>M2</Name><Origin><Source>GeometricFeature</Source><FeatureName>circular curve 838</FeatureName></Origin><PrimaryAxis><DefinedDirection>+Z</DefinedDirection><Source>ReferenceFrame</Source><SourceDirection>+Z</SourceDirection><FeatureName></FeatureName></PrimaryAxis><SecondaryAxis><DefinedDirection>+X</DefinedDirection><Source>ReferenceFrame</Source><SourceDirection>+X</SourceDirection><FeatureName></FeatureName></SecondaryAxis></Value></Frame><Frame><Id>Frame3</Id><Value><Name>M1</Name><Origin><Source>GeometricFeature</Source><FeatureName>circular curve 1634</FeatureName></Origin><PrimaryAxis><DefinedDirection>+Z</DefinedDirection><Source>ReferenceFrame</Source><SourceDirection>+Z</SourceDirection><FeatureName></FeatureName></PrimaryAxis><SecondaryAxis><DefinedDirection>+Y</DefinedDirection><Source>ReferenceFrame</Source><SourceDirection>+X</SourceDirection><FeatureName></FeatureName></SecondaryAxis></Value></Frame><Frame><Id>Frame4</Id><Value><Name>M3</Name><Origin><Source>GeometricFeature</Source><FeatureName>circular curve 1236</FeatureName></Origin><PrimaryAxis><DefinedDirection>+Z</DefinedDirection><Source>ReferenceFrame</Source><SourceDirection>+Z</SourceDirection><FeatureName></FeatureName></PrimaryAxis><SecondaryAxis><DefinedDirection>+X</DefinedDirection><Source>ReferenceFrame</Source><SourceDirection>+X</SourceDirection><FeatureName></FeatureName></SecondaryAxis></Value></Frame><Frame><Id>Frame5</Id><Value><Name>M4</Name><Origin><Source>GeometricFeature</Source><FeatureName>circular curve 2038</FeatureName></Origin><PrimaryAxis><DefinedDirection>+Z</DefinedDirection><Source>ReferenceFrame</Source><SourceDirection>+Z</SourceDirection><FeatureName></FeatureName></PrimaryAxis><SecondaryAxis><DefinedDirection>+X</DefinedDirection><Source>ReferenceFrame</Source><SourceDirection>+X</SourceDirection><FeatureName></FeatureName></SecondaryAxis></Value></Frame></Frames>  GraphicType=FromGeometry  MarkerShape=Sphere  MarkerSize=10  GraphicVisPropType=SimpleVisualProperties  GraphicDiffuseColor=[0.5 0.5 0.5]  GraphicSpecularColor=[0.5 0.5 0.5 1.0]  GraphicAmbientColor=[0.15 0.15 0.15 1.0]  GraphicEmissiveColor=[0.0 0.0 0.0 1.0]  GraphicShininess=75  GraphicOpacity=1.0
  Clock : Clock
  Contact Detector : Subsystem  Commented=on
      settings: PortSchema="{\"entries\":[{\"content\":{\"sides\":[{\"content\":{\"connectorIds\":[\"LConn1\",\"In1\",\"In2\"]},\"type\":\"ConnectorPlacement.EquallySpacedRectSide\",\"uuid\":\"73a6758d-74b0-4dfa-ae59-8f1544b47e52\"},{\"content\":{\"connectorIds\":[\"RConn1\"],\"side\":\"RIGHT\"},\"type\":\"ConnectorPlacement.EquallySpacedRectSide\",\"uuid\":\"cda79cee-8790-4a48-af2a-c8e672ccd871\"},{\"content\":{\"connectorIds\":[],\"side\":\"TOP\"},\"type\":\"ConnectorPlacement.EquallySpacedRectSide\",\"uuid\":\"3568e893-e479-4ecf-b205-b5b750c24788\"}]},\"type\":\"ConnectorPlacement.EquallySpacedConnector\",\"uuid\":\"7addec4e-c0c3-4372-b547-1236ed1106f4\"}],\"packageUris\":[\"http://schema.mathworks.com/mf0/Connector/R2020b\"],\"version\":\"1.0\"}"
  Demux : Demux  Outputs=3
  Infinite Plane : sm_lib/Curves and Surfaces/Infinite Plane  GraphicType=Rectangle  GraphicPlaneWidth=10  GraphicPlaneWidthUnits=m  GraphicPlaneHeight=10  GraphicPlaneHeightUnits=m  GraphicVisPropType=SimpleVisualProperties  GraphicDiffuseColor=[1 0.07451 0.651]  GraphicOpacity=0.25  GraphicSpecularColor=[0.5 0.5 0.5 1.0]  GraphicAmbientColor=[0.15 0.15 0.15 1.0]  GraphicEmissiveColor=[0.0 0.0 0.0 1.0]  GraphicShininess=75
  "Propeller 1 " : sm_lib/Body Elements/File Solid  ExtGeomFileName=SolidFiles\propeller_blade_black.STEP  UnitType=FromFile  ExtGeomFileUnits=m  StepReaderType=HEX  ExportConvexHullGeometry=off  InertiaType=Custom  Mass=0.00001  MassUnits=kg  CenterOfMass=[0 0 0]  CenterOfMassUnits=m  MomentsOfInertia=[1e-12 1e-12 1e-12]  MomentsOfInertiaUnits=kg*m^2  ProductsOfInertia=[0 0 0]  ProductsOfInertiaUnits=kg*m^2  BasedOnType=Mass  Density=1000  DensityUnits=kg/m^3  DoExposeReferenceFrame=off  SerializedFrames=<Frames><Frame><Id>Frame1</Id><Value><Name>F1</Name><Origin><Source>CenterOfMassFrame</Source><FeatureName></FeatureName></Origin><PrimaryAxis><DefinedDirection>-X</DefinedDirection><Source>ReferenceFrame</Source><SourceDirection>+Z</SourceDirection><FeatureName></FeatureName></PrimaryAxis><SecondaryAxis><DefinedDirection>+Y</DefinedDirection><Source>ReferenceFrame</Source><SourceDirection>+X</SourceDirection><FeatureName></FeatureName></SecondaryAxis></Value></Frame></Frames>  GraphicType=FromGeometry  MarkerShape=Sphere  MarkerSize=10  GraphicVisPropType=SimpleVisualProperties  GraphicDiffuseColor=[1.0 0.2 0.2]  GraphicSpecularColor=[0.5 0.5 0.5 1.0]  GraphicAmbientColor=[0.15 0.15 0.15 1.0]  GraphicEmissiveColor=[0.0 0.0 0.0 1.0]  GraphicShininess=75  GraphicOpacity=1.0
  Propeller 2 : sm_lib/Body Elements/File Solid  ExtGeomFileName=SolidFiles\propeller_blade_black.STEP  UnitType=FromFile  ExtGeomFileUnits=m  StepReaderType=HEX  ExportConvexHullGeometry=off  InertiaType=Custom  Mass=0.00001  MassUnits=kg  CenterOfMass=[0 0 0]  CenterOfMassUnits=m  MomentsOfInertia=[1e-12 1e-12 1e-12]  MomentsOfInertiaUnits=kg*m^2  ProductsOfInertia=[0 0 0]  ProductsOfInertiaUnits=kg*m^2  BasedOnType=Mass  Density=1000  DensityUnits=kg/m^3  DoExposeReferenceFrame=off  SerializedFrames=<Frames><Frame><Id>Frame1</Id><Value><Name>F1</Name><Origin><Source>CenterOfMassFrame</Source><FeatureName></FeatureName></Origin><PrimaryAxis><DefinedDirection>-X</DefinedDirection><Source>ReferenceFrame</Source><SourceDirection>+Z</SourceDirection><FeatureName></FeatureName></PrimaryAxis><SecondaryAxis><DefinedDirection>+Y</DefinedDirection><Source>ReferenceFrame</Source><SourceDirection>+X</SourceDirection><FeatureName></FeatureName></SecondaryAxis></Value></Frame></Frames>  GraphicType=FromGeometry  MarkerShape=Sphere  MarkerSize=10  GraphicVisPropType=SimpleVisualProperties  GraphicDiffuseColor=[1.0 0.2 0.2]  GraphicSpecularColor=[0.5 0.5 0.5 1.0]  GraphicAmbientColor=[0.15 0.15 0.15 1.0]  GraphicEmissiveColor=[0.0 0.0 0.0 1.0]  GraphicShininess=75  GraphicOpacity=1.0
  Propeller 3 : sm_lib/Body Elements/File Solid  ExtGeomFileName=SolidFiles\propeller_blade_black.STEP  UnitType=FromFile  ExtGeomFileUnits=m  StepReaderType=HEX  ExportConvexHullGeometry=off  InertiaType=Custom  Mass=0.00001  MassUnits=kg  CenterOfMass=[0 0 0]  CenterOfMassUnits=m  MomentsOfInertia=[1e-12 1e-12 1e-12]  MomentsOfInertiaUnits=kg*m^2  ProductsOfInertia=[0 0 0]  ProductsOfInertiaUnits=kg*m^2  BasedOnType=Mass  Density=1000  DensityUnits=kg/m^3  DoExposeReferenceFrame=off  SerializedFrames=<Frames><Frame><Id>Frame1</Id><Value><Name>F1</Name><Origin><Source>CenterOfMassFrame</Source><FeatureName></FeatureName></Origin><PrimaryAxis><DefinedDirection>-X</DefinedDirection><Source>ReferenceFrame</Source><SourceDirection>+Z</SourceDirection><FeatureName></FeatureName></PrimaryAxis><SecondaryAxis><DefinedDirection>+Y</DefinedDirection><Source>ReferenceFrame</Source><SourceDirection>+X</SourceDirection><FeatureName></FeatureName></SecondaryAxis></Value></Frame></Frames>  GraphicType=FromGeometry  MarkerShape=Sphere  MarkerSize=10  GraphicVisPropType=SimpleVisualProperties  GraphicDiffuseColor=[1.0 0.2 0.2]  GraphicSpecularColor=[0.5 0.5 0.5 1.0]  GraphicAmbientColor=[0.15 0.15 0.15 1.0]  GraphicEmissiveColor=[0.0 0.0 0.0 1.0]  GraphicShininess=75  GraphicOpacity=1.0
  Propeller 4 : sm_lib/Body Elements/File Solid  ExtGeomFileName=SolidFiles\propeller_blade_black.STEP  UnitType=FromFile  ExtGeomFileUnits=m  StepReaderType=HEX  ExportConvexHullGeometry=off  InertiaType=Custom  Mass=0.00001  MassUnits=kg  CenterOfMass=[0 0 0]  CenterOfMassUnits=m  MomentsOfInertia=[1e-12 1e-12 1e-12]  MomentsOfInertiaUnits=kg*m^2  ProductsOfInertia=[0 0 0]  ProductsOfInertiaUnits=kg*m^2  BasedOnType=Mass  Density=1000  DensityUnits=kg/m^3  DoExposeReferenceFrame=off  SerializedFrames=<Frames><Frame><Id>Frame1</Id><Value><Name>F1</Name><Origin><Source>CenterOfMassFrame</Source><FeatureName></FeatureName></Origin><PrimaryAxis><DefinedDirection>-X</DefinedDirection><Source>ReferenceFrame</Source><SourceDirection>+Z</SourceDirection><FeatureName></FeatureName></PrimaryAxis><SecondaryAxis><DefinedDirection>+Y</DefinedDirection><Source>ReferenceFrame</Source><SourceDirection>+X</SourceDirection><FeatureName></FeatureName></SecondaryAxis></Value></Frame></Frames>  GraphicType=FromGeometry  MarkerShape=Sphere  MarkerSize=10  GraphicVisPropType=SimpleVisualProperties  GraphicDiffuseColor=[1.0 0.2 0.2]  GraphicSpecularColor=[0.5 0.5 0.5 1.0]  GraphicAmbientColor=[0.15 0.15 0.15 1.0]  GraphicEmissiveColor=[0.0 0.0 0.0 1.0]  GraphicShininess=75  GraphicOpacity=1.0
  Ramp : simulink/Sources/Ramp  slope=-8  start=0  InitialOutput=0
  Ramp1 : simulink/Sources/Ramp  slope=8  start=0  InitialOutput=0
  Ramp2 : simulink/Sources/Ramp  slope=8  start=0  InitialOutput=0
  Ramp3 : simulink/Sources/Ramp  slope=-8  start=0  InitialOutput=0
  Revolute Joint{,1..3} (4 alike) : sm_lib/Joints/Revolute Joint  JointMode=Normal  SenseConstraintForce=off  SenseConstraintForceX=off  SenseConstraintForceY=off  SenseConstraintForceZ=off  SenseConstraintTorque=off  SenseConstraintTorqueX=off  SenseConstraintTorqueY=off  SenseConstraintTorqueZ=off  SenseTotalForce=off  SenseTotalForceX=off  SenseTotalForceY=off  SenseTotalForceZ=off  SenseTotalTorque=off  SenseTotalTorqueX=off  SenseTotalTorqueY=off  SenseTotalTorqueZ=off  CompositeWrenchDir=FollowerOnBase  CompositeWrenchFrame=BaseFrame  EquilibriumPosition=0  EquilibriumPositionUnits=deg  SpringStiffness=0  SpringStiffnessUnits=N*m/deg  DampingCoefficient=0  DampingCoefficientUnits=N*m/(deg/s)  TorqueActuationMode=ComputedTorque  MotionActuationMode=InputMotion  SensePosition=off  SenseVelocity=off  SenseAcceleration=off  SenseTorqueForce=off  SenseLowerLimitTorqueForce=off  SenseUpperLimitTorqueForce=off  LowerLimitSpecify=off  LowerLimitBound=-90  LowerLimitBoundUnits=deg  LowerLimitStiffness=1e4  LowerLimitStiffnessUnits=N*m/deg  LowerLimitDamping=10  LowerLimitDampingUnits=N*m/(deg/s)  LowerLimitTransitionRegionWidth=0.1  LowerLimitTransitionRegionWidthUnits=deg  UpperLimitSpecify=off  UpperLimitBound=90  UpperLimitBoundUnits=deg  UpperLimitStiffness=1e4  UpperLimitStiffnessUnits=N*m/deg  UpperLimitDamping=10  UpperLimitDampingUnits=N*m/(deg/s)  UpperLimitTransitionRegionWidth=0.1  UpperLimitTransitionRegionWidthUnits=deg  PositionTargetSpecify=off  PositionTargetPriority=High  PositionTargetValue=0  PositionTargetValueUnits=deg  VelocityTargetSpecify=off  VelocityTargetPriority=High  VelocityTargetValue=0  VelocityTargetValueUnits=deg/s
  Simulink-PS Converter{6..9} (4 alike) : nesl_utility/Simulink-PS Converter  PhysicalDomain=network_engine_domain  SubClassName=ps_input  LeftPortType=input  RightPortType=output  PseudoPeriodic=off  Frequencies=[]  NoiseDistribution=none  NoiseParameters=[]  Unit=1  AffineConversion=off  FilteringAndDerivatives=filter  SimscapeFilterOrder=2  InputFilterTimeConstant=0.1  UdotUserProvided=0
  Spatial Contact Force : sm_lib/Forces and Torques/Spatial Contact Force  Commented=on  SenseContactBaseRotation=off  SenseContactBaseTranslation=off  CoefficientOfDynamicFriction=0.3  CoefficientOfStaticFriction=0.5  NormalDamping=1e3  NormalDampingUnits=N/(m/s)  SenseContactSignal=off  NormalStiffness=1e6  NormalStiffnessUnits=N/m  FrictionalCriticalVelocity=1e-3  FrictionalCriticalVelocityUnits=m/s  ZeroCrossDetectContactStartAndEnd=off  SenseContactFollowerRotation=off  SenseContactFollowerTranslation=off  FrictionType=SmoothStickSlip  SenseFrictionalForceMagnitude=off  SenseNormalForceMagnitude=off  NormalForceType=SmoothSpringDamper  SenseNormalVelocity=off  SenseSeparationDistance=off  SenseTangentialVelocity=off  NormalTransitionRegionWidth=1e-4  NormalTransitionRegionWidthUnits=m
  Terminator : Terminator
  To Workspace : ToWorkspace  VariableName=time  SampleTime=-1
      settings: Save2DSignal=2-D array (concatenate along first dimension)
  base : PMIOPort  Side=Left
  motion : PMIOPort  Port=2  Side=Left
  wires:
  Ramp1/1 -> Simulink-PS Converter7/1
  Ramp3/1 -> Simulink-PS Converter9/1
  Ramp2/1 -> Simulink-PS Converter8/1
  Ramp/1 -> Simulink-PS Converter6/1
  Demux/3 -> Terminator/1
  lambda/1 -> Demux/1
  Clock/1 -> To Workspace/1
  connections:
  Simulink-PS Converter9/RConn1 -- Revolute Joint3/LConn2
  Simulink-PS Converter6/RConn1 -- Revolute Joint/LConn2
  Revolute Joint1/RConn1 -- Propeller 4/LConn1
  Simulink-PS Converter7/RConn1 -- Revolute Joint1/LConn2
  Revolute Joint1/LConn1 -- Body/LConn3
  Simulink-PS Converter8/RConn1 -- Revolute Joint2/LConn2
  Revolute Joint2/RConn1 -- Propeller 2/LConn1
  Body/LConn1 -- motion/RConn1
  Body/RConn2 -- Revolute Joint3/LConn1
  Body/LConn2 -- Revolute Joint/LConn1
  Body/RConn1 -- Revolute Joint2/LConn1
  Revolute Joint3/RConn1 -- Propeller 3/LConn1
  Revolute Joint/RConn1 -- "Propeller 1 "/LConn1
  base/RConn1 -- Infinite Plane/LConn1
  Body/RConn3 -- Spatial Contact Force/RConn1
  Infinite Plane/RConn1 -- Spatial Contact Force/LConn1

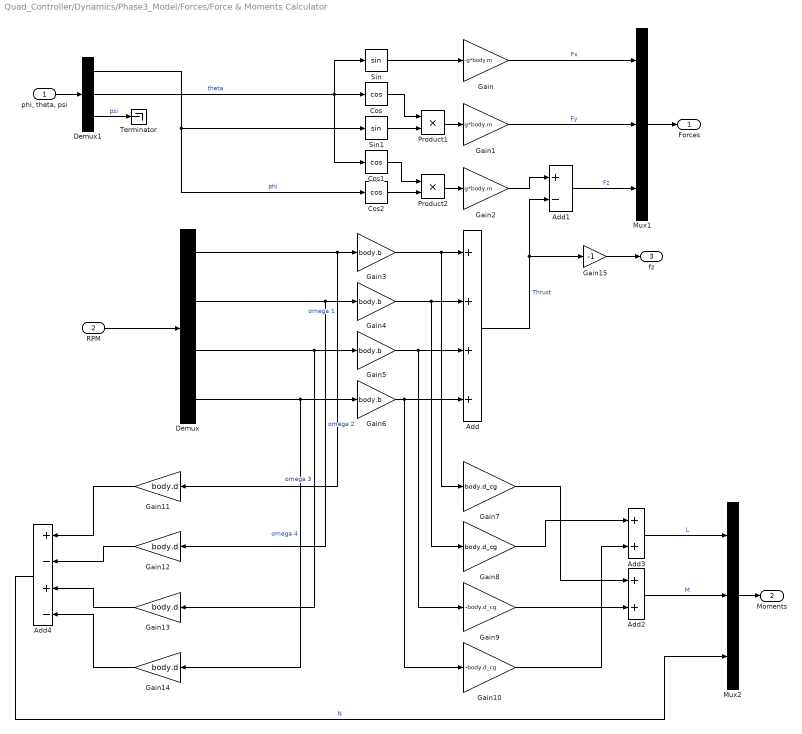
== system Quad_Controller/Dynamics/Phase3_Model/Forces/Force & Moments Calculator ==
  "phi, theta, psi" : Inport
  RPM : Inport  Port=2
  Add : Sum  Inputs=++++
  Add1 : Sum  Inputs=+-
  Add2 : Sum
  Add3 : Sum
  Add4 : Sum  Inputs=+-+-
  Cos : Trigonometry  Operator=cos
  Cos1 : Trigonometry  Operator=cos
  Cos2 : Trigonometry  Operator=cos
  Demux : Demux
  Demux1 : Demux  Outputs=3
  Gain : Gain  Gain=-g*body.m
  Gain1 : Gain  Gain=g*body.m
  Gain10 : Gain  Gain=-body.d_cg
  Gain{11..14} (4 alike) : Gain  Gain=body.d
  Gain15 : Gain  Gain=-1
  Gain2 : Gain  Gain=g*body.m
  Gain{3..6} (4 alike) : Gain  Gain=body.b
  Gain7 : Gain  Gain=body.d_cg
  Gain8 : Gain  Gain=body.d_cg
  Gain9 : Gain  Gain=-body.d_cg
  Mux1 : Mux  Inputs=3
  Mux2 : Mux  Inputs=3
  Product1 : Product
  Product2 : Product
  Sin : Trigonometry
  Sin1 : Trigonometry
  Terminator : Terminator
  Forces : Outport
  Moments : Outport  Port=2
  fz : Outport  Port=3
  wires:
  Cos2/1 -> Product2/2
  Cos1/1 -> Product2/1
  Gain1/1 -> Mux1/2  "Fy"
  Demux/3 -> Gain13/1, Gain5/1  "omega 3"
  Gain5/1 -> Gain9/1, Add/3
  Gain2/1 -> Add1/1
  Demux1/1 -> Sin1/1, Cos2/1  "phi"
  Add3/1 -> Mux2/1  "L"
  Gain4/1 -> Gain8/1, Add/2
  Gain6/1 -> Gain10/1, Add/4
  Gain3/1 -> Gain7/1, Add/1
  Demux/2 -> Gain12/1, Gain4/1  "omega 2"
  Gain9/1 -> Add2/2
  Sin1/1 -> Product1/2
  Gain/1 -> Mux1/1  "Fx"
  Add2/1 -> Mux2/2  "M"
  Gain13/1 -> Add4/3
  Demux/1 -> Gain11/1, Gain3/1  "omega 1"
  Demux1/2 -> Sin/1, Cos1/1, Cos/1  "theta"
  Gain7/1 -> Add2/1
  Gain14/1 -> Add4/4
  Demux/4 -> Gain14/1, Gain6/1  "omega 4"
  Cos/1 -> Product1/1
  Gain12/1 -> Add4/2
  Add/1 -> Gain15/1, Add1/2  "Thrust"
  Add4/1 -> Mux2/3  "N"
  Mux2/1 -> Moments/1
  Gain11/1 -> Add4/1
  Sin/1 -> Gain/1
  Product1/1 -> Gain1/1
  Add1/1 -> Mux1/3  "Fz"
  Gain8/1 -> Add3/1
  RPM/1 -> Demux/1
  Gain10/1 -> Add3/2
  Product2/1 -> Gain2/1
  Mux1/1 -> Forces/1
  "phi, theta, psi"/1 -> Demux1/1
  Demux1/3 -> Terminator/1  "psi"
  Gain15/1 -> fz/1

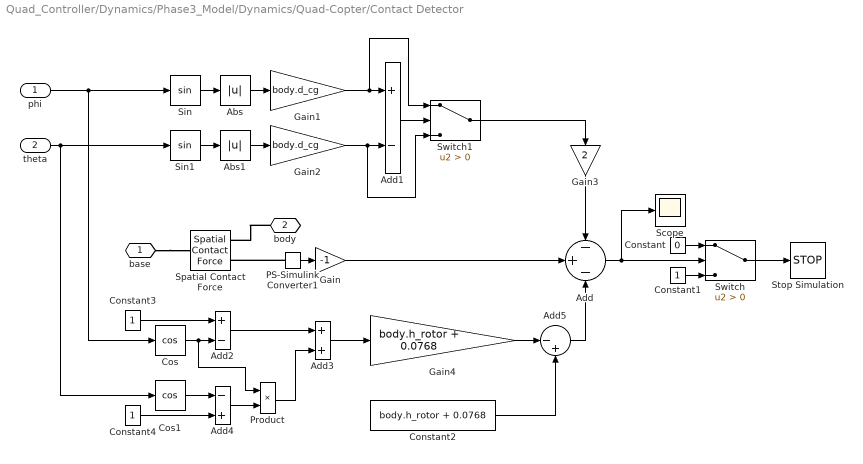
== system Quad_Controller/Dynamics/Phase3_Model/Dynamics/Quad-Copter/Contact Detector ==
  phi : Inport
  theta : Inport  Port=2
  Abs : Abs  SaturateOnIntegerOverflow=off
  Abs1 : Abs  SaturateOnIntegerOverflow=off
  Add : Sum  Inputs=-+-
  Add1 : Sum  Inputs=+-
  Add2 : Sum  Inputs=+-
  Add3 : Sum
  Add4 : Sum  Inputs=-+
  Add5 : Sum  Inputs=|-+
  Constant : Constant  Value=0
  Constant1 : Constant
  Constant2 : Constant  Value=body.h_rotor + 0.0768
  Constant3 : Constant
  Constant4 : Constant
  Cos : Trigonometry  Operator=cos
  Cos1 : Trigonometry  Operator=cos
  Gain : Gain  Gain=-1
  Gain1 : Gain  Gain=body.d_cg
  Gain2 : Gain  Gain=body.d_cg
  Gain3 : Gain  Gain=2
  Gain4 : Gain  Gain=body.h_rotor + 0.0768
  PS-Simulink Converter1 : nesl_utility/PS-Simulink Converter  PhysicalDomain=network_engine_domain  SubClassName=ps_output  LeftPortType=input  RightPortType=output  PseudoPeriodic=off  Frequencies=[]  VectorFormat=inherit  Unit=inherit  AffineConversion=off
  Product : Product
  Scope : Scope
  Sin : Trigonometry
  Sin1 : Trigonometry
  Spatial Contact Force : sm_lib/Forces and Torques/Spatial Contact Force  SenseContactBaseRotation=off  SenseContactBaseTranslation=off  CoefficientOfDynamicFriction=0.3  CoefficientOfStaticFriction=0.5  NormalDamping=1e3  NormalDampingUnits=N/(m/s)  SenseContactSignal=off  NormalStiffness=1e6  NormalStiffnessUnits=N/m  FrictionalCriticalVelocity=1e-3  FrictionalCriticalVelocityUnits=m/s  ZeroCrossDetectContactStartAndEnd=off  SenseContactFollowerRotation=off  SenseContactFollowerTranslation=off  FrictionType=SmoothStickSlip  SenseFrictionalForceMagnitude=off  SenseNormalForceMagnitude=off  NormalForceType=SmoothSpringDamper  SenseNormalVelocity=off  SenseSeparationDistance=on  SenseTangentialVelocity=off  NormalTransitionRegionWidth=1e-4  NormalTransitionRegionWidthUnits=m
  Stop Simulation : Stop
  Switch : Switch  Criteria=u2 > Threshold  SaturateOnIntegerOverflow=off  InputSameDT=off
  Switch1 : Switch  Criteria=u2 > Threshold  SaturateOnIntegerOverflow=off  InputSameDT=off
  base : PMIOPort  Side=Left
  body : PMIOPort  Port=2  Side=Right
  wires:
  Constant1/1 -> Switch/3
  PS-Simulink Converter1/1 -> Gain/1
  Constant/1 -> Switch/1
  Add/1 -> Scope/1, Switch/2
  phi/1 -> Cos/1, Sin/1
  theta/1 -> Cos1/1, Sin1/1
  Gain2/1 -> Switch1/3, Add1/2
  Gain1/1 -> Switch1/1, Add1/1
  Add1/1 -> Switch1/2
  Sin/1 -> Abs/1
  Abs/1 -> Gain1/1
  Sin1/1 -> Abs1/1
  Abs1/1 -> Gain2/1
  Gain/1 -> Add/2
  Switch1/1 -> Gain3/1
  Gain3/1 -> Add/1
  Cos/1 -> Product/1, Add2/2
  Constant3/1 -> Add2/1
  Add2/1 -> Add3/1
  Cos1/1 -> Add4/1
  Constant4/1 -> Add4/2
  Add4/1 -> Product/2
  Product/1 -> Add3/2
  Add3/1 -> Gain4/1
  Gain4/1 -> Add5/1
  Constant2/1 -> Add5/2
  Add5/1 -> Add/3
  Switch/1 -> Stop Simulation/1
  connections:
  body/RConn1 -- Spatial Contact Force/RConn1
  PS-Simulink Converter1/LConn1 -- Spatial Contact Force/RConn2
  base/RConn1 -- Spatial Contact Force/LConn1

== matlab function Quad_Controller/Dynamics/Phase3_Model/Dynamics/MATLAB Function ==
  data: lambda input; omega output; phi_d input; theta_d input; psi_d input
function omega = fcn(lambda, phi_d, theta_d, psi_d)
    phi = lambda(1); theta = lambda(2); 

    pqr = [1 0 -sin(theta);
             0 cos(phi) sin(phi)*cos(theta);
             0 -sin(phi) cos(phi)*cos(theta)]*[phi_d; theta_d; psi_d];

    omega = [pqr(1) pqr(2) pqr(3)];
end

== matlab function Quad_Controller/Dynamics/Phase3_Model/Forces/MATLAB Function ==
  data: fz input; fxG output; lambda input; fyG output; fzG output
function [fxG, fyG, fzG] = fcn(fz, lambda)
    phi = lambda(1); theta = lambda(2); psi = lambda(3);

    fxG = fz*(cos(phi)*sin(theta)*cos(psi)+sin(phi)*sin(psi));
    fyG = fz*(cos(phi)*sin(theta)*sin(psi)-sin(phi)*cos(psi));
    fzG = fz*(cos(phi)*cos(theta));
end

== matlab function Quad_Controller/Dynamics/Phase3_Model/Dynamics/MATLAB Function1 ==
  data: lambda input; Vb output; Vx input; Vy input; Vz input
function Vb = fcn(lambda, Vx, Vy, Vz)
    phi = lambda(1); theta = lambda(2); 

    V = [1 0 -sin(theta);
             0 cos(phi) sin(phi)*cos(theta);
             0 -sin(phi) cos(phi)*cos(theta)]*[Vx; Vy; Vz];

    Vb = [V(1) V(2) V(3)];
end
